simulink model "motor_sensorless"  (R2020a)
settings: Solver=FixedStepDiscrete  StartTime=0.0  StopTime=inf  FixedStep=ts  RelTol=1e-3
values from neighbouring files (symbols this model uses):
  adgain_and_ivscale = round(0.33*1.56*4096/3.3*SC_SCALE/IV_SCALE)    [def_param.m]
  cos23z = round(cos(2.0/3.0*pi)*sqrt(2.0/3.0)*SC_SCALE)    [def_param.m]
  cos43z = round(cos(4.0/3.0*pi)*sqrt(2.0/3.0)*SC_SCALE)    [def_param.m]
  COUNT2RPM = round(FS/SC_SCALE*60/7)    [def_param.m]
  DUTY2VOLT = round(VCC*IV_SCALE/MAX_PWM_DUTY)    [def_param.m]
  FF_CURRENT = 1500    [def_param.m]
  FS = 20000    [def_param.m]
  iKi_pll = round(1/Ki_pll)    [def_param.m]
  iKp_curr_d = iKp_curr    [def_param.m]
  iKp_curr_q = iKp_curr    [def_param.m]
  iKp_pll = round(1/Kp_pll)    [def_param.m]
  Ki_curr_d = Ki_curr    [def_param.m]
  Ki_curr_q = Ki_curr    [def_param.m]
  Kp_velo = 5    [def_param.m]
  Ra_scale = round(Ra*SC_SCALE)    [def_param.m]
  SC_SCALE = 32768    [def_param.m]
  sin23z = round(sin(2.0/3.0*pi)*sqrt(2.0/3.0)*SC_SCALE)    [def_param.m]
  sin43z = round(sin(4.0/3.0*pi)*sqrt(2.0/3.0)*SC_SCALE)    [def_param.m]
  sqrt23 = round(sqrt(2.0/3.0)*SC_SCALE)    [def_param.m]
libraries: simulink x2, arduinolib x1
settings Model: SimulationMode=external  SILPILModeSetting=veronly  ExtModeTrigDuration=1  Creator=hirata  LastModifiedBy=hirata
settings DataIOCC: SaveOutput=off  SignalLogging=off  DSMLogging=off  SaveTime=off  ReturnWorkspaceOutputs=off
settings OptimizationCC: EnhancedBackFolding=on  PassReuseOutputArgsAs=Individual arguments  ZeroExternalMemoryAtStartup=off  ZeroInternalMemoryAtStartup=off  MaxStackSize=64  OptimizeBlockOrder=speed  DifferentSizesBufferReuse=on  OptimizationCustomize=off  EfficientTunableParamExpr=on
settings DebuggingCC: MultiTaskDSMMsg=none  ParameterTunabilityLossMsg=error
settings HardwareCC: ProdBitPerPointer=32  ProdBitPerSizeT=32  ProdBitPerPtrDiffT=32  ProdLargestAtomicInteger=Long  ProdLargestAtomicFloat=Double  ProdWordSize=32  ProdHWDeviceType=ARM Compatible->ARM Cortex  UseEmbeddedCoderFeatures=off  UseSimulinkCoderFeatures=off
settings SFSimCC: MATLABDynamicMemAlloc=off
settings RTWCC: SystemTargetFile=ert.tlc  HardwareBoard=Arduino Due  TLCOptions=-aInlineSetEventsForThisBaseRateFcn=TLC_FALSE -aSuppressMultiTaskScheduler=TLC_FALSE -aRateBasedStepFcn=1  TemplateMakefile=ert_default_tmf  Toolchain=Arduino ARM  BuildConfiguration=Faster Runs
settings CodeAppCC: ForceParamTrailComments=on  IgnoreCustomStorageClasses=off  OperatorAnnotations=on  SimulinkDataObjDesc=on  SFDataObjDesc=on  InsertBlockDesc=on
settings ERTTargetCC: SupportContinuousTime=on  SupportNonInlinedSFcns=on  SupportVariableSizeSignals=on  ExtModeStaticAllocSize=24576

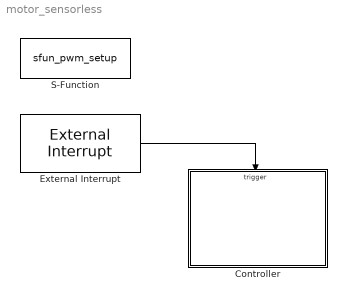
== system motor_sensorless ==
  Controller : Subsystem
  External Interrupt : arduinolib/External Interrupt  Pin=2  PullUp=off  Mode=RISING  InterruptSimulationInput=off
      settings: SourceProductBaseCode=ARDUINO
  S-Function : S-Function  FunctionName=sfun_pwm_setup  SFunctionDeploymentMode=off  EnableBusSupport=off
  wires:
  External Interrupt/1 -> Controller/Trigger

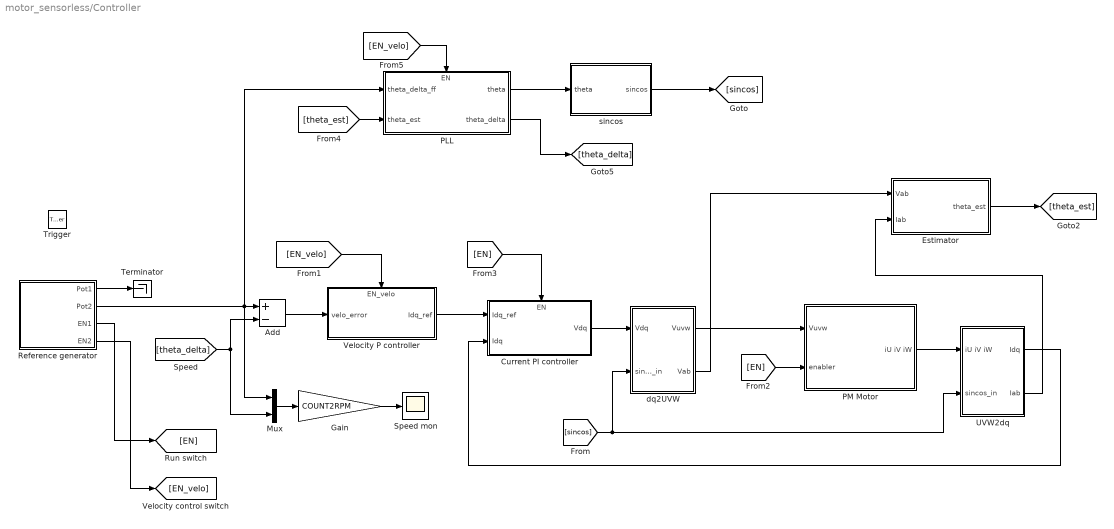
== system motor_sensorless/Controller ==
  Trigger : TriggerPort  TriggerType=function-call  VariantControl=Variant  PortDimensions=1
  Add : Sum  Inputs=+-
  Current PI controller : Subsystem
      settings: PortSchema="{\"entries\":[{\"content\":{\"sides\":[{\"content\":{\"connectorIds\":[\"In1\",\"In2\"]},\"type\":\"ConnectorPlacement.EquallySpacedRectSide\",\"uuid\":\"51bdd515-79d8-44f5-b943-076c1de5691d\"},{\"content\":{\"connectorIds\":[\"Out1\"],\"side\":\"RIGHT\"},\"type\":\"ConnectorPlacement.EquallySpacedRectSide\",\"uuid\":\"02ded229-b196-46a0-b1f1-559478ee2a5f\"},{\"content\":{\"connectorIds\":[\"In3\"],\"side\":\"TOP\"},\"type\":\"ConnectorPlacement.EquallySpacedRectSide\",\"uuid\":\"45d1ca2d-8d37-43f9-8461-d73100be391d\"}]},\"type\":\"ConnectorPlacement.EquallySpacedConnector\",\"uuid\":\"0325882b-c054-4400-b3a7-6975fb1af6b3\"}],\"packageUris\":[\"http://schema.mathworks.com/mf0/Connector/19700101\"],\"version\":\"1.0\"}"
  Estimator : Subsystem
  Gain : Gain  Gain=COUNT2RPM  ParamDataTypeStr=int32  OutDataTypeStr=int32
  Mux : Mux  Inputs=2
  PLL : Subsystem
      settings: PortSchema="{\"entries\":[{\"content\":{\"sides\":[{\"content\":{\"connectorIds\":[\"In1\",\"In2\"]},\"type\":\"ConnectorPlacement.EquallySpacedRectSide\",\"uuid\":\"c1279200-642a-4817-bff2-49f1fc45cae9\"},{\"content\":{\"connectorIds\":[\"Out1\",\"Out2\"],\"side\":\"RIGHT\"},\"type\":\"ConnectorPlacement.EquallySpacedRectSide\",\"uuid\":\"60873783-c9ec-4a70-a078-e4f3fd5ab03e\"},{\"content\":{\"connectorIds\":[\"In3\"],\"side\":\"TOP\"},\"type\":\"ConnectorPlacement.EquallySpacedRectSide\",\"uuid\":\"f4a28572-fe2d-4ee0-bb44-94978f18e4bd\"}]},\"type\":\"ConnectorPlacement.EquallySpacedConnector\",\"uuid\":\"bfaa0106-d9f2-4ecc-a1fc-3a6fb0b4180b\"}],\"packageUris\":[\"http://schema.mathworks.com/mf0/Connector/19700101\"],\"version\":\"1.0\"}"
  PM Motor : Subsystem
  Reference generator : Subsystem
  Speed mon : Scope
  Terminator : Terminator
  UVW2dq : Subsystem
  Velocity P controller : Subsystem
      settings: PortSchema="{\"entries\":[{\"content\":{\"sides\":[{\"content\":{\"connectorIds\":[\"In1\"]},\"type\":\"ConnectorPlacement.EquallySpacedRectSide\",\"uuid\":\"ec985efa-ceb5-40b6-8715-0b6e8d029389\"},{\"content\":{\"connectorIds\":[\"Out1\"],\"side\":\"RIGHT\"},\"type\":\"ConnectorPlacement.EquallySpacedRectSide\",\"uuid\":\"25d854cf-6db0-4509-b167-323bc7ab570a\"},{\"content\":{\"connectorIds\":[\"In2\"],\"side\":\"TOP\"},\"type\":\"ConnectorPlacement.EquallySpacedRectSide\",\"uuid\":\"c6db0138-fa8b-40e2-8338-1c9cb4bbe622\"}]},\"type\":\"ConnectorPlacement.EquallySpacedConnector\",\"uuid\":\"967c00c6-7ce0-4d1f-a7f0-366bbe0d8034\"}],\"packageUris\":[\"http://schema.mathworks.com/mf0/Connector/19700101\"],\"version\":\"1.0\"}"
  dq2UVW : Subsystem
  sincos : Subsystem
  wires:
  dq2UVW/1(Vuvw) -> PM Motor/1(Vuvw)
  [sincos] -> dq2UVW/2(sincos_in), UVW2dq/2(sincos_in)
  PM Motor/1(iU iV iW) -> UVW2dq/1(iU iV iW)
  UVW2dq/1(Idq) -> Current PI controller/2(Idq)
  [EN] -> PM Motor/2(enabler)
  Current PI controller/1(Vdq) -> dq2UVW/1(Vdq)
  [EN] -> Current PI controller/3(EN)
  dq2UVW/2(Vab) -> Estimator/1(Vab)
  UVW2dq/2(Iab) -> Estimator/2(Iab)
  Estimator/1(theta_est) -> [theta_est]
  [theta_est] -> PLL/2(theta_est)
  [EN_velo] -> PLL/3(EN)
  PLL/1(theta) -> sincos/1(theta)
  sincos/1(sincos) -> [sincos]
  Add/1 -> Velocity P controller/1(velo_error)
  [EN_velo] -> Velocity P controller/2(EN_velo)
  Velocity P controller/1(Idq_ref) -> Current PI controller/1(Idq_ref)
  PLL/2(theta_delta) -> [theta_delta]
  [theta_delta] -> Mux/2, Add/2
  Reference generator/2(Pot2) -> Mux/1, PLL/1(theta_delta_ff), Add/1
  Reference generator/3(EN1) -> [EN]
  Reference generator/4(EN2) -> [EN_velo]
  Mux/1 -> Gain/1
  Reference generator/1(Pot1) -> Terminator/1
  Gain/1 -> Speed mon/1

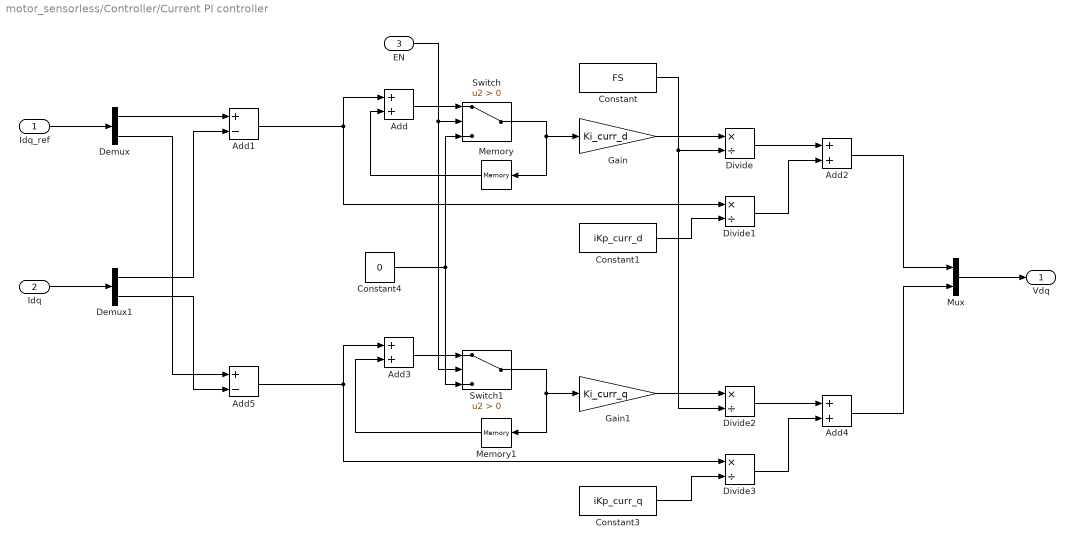
== system motor_sensorless/Controller/Current PI controller ==
  Idq_ref : Inport
  Idq : Inport  Port=2
  EN : Inport  Port=3
  Add{,2..4} (4 alike) : Sum
  Add1 : Sum  Inputs=+-
  Add5 : Sum  Inputs=+-
  Constant : Constant  Value=FS  OutDataTypeStr=int32
  Constant1 : Constant  Value=iKp_curr_d  OutDataTypeStr=int32
  Constant3 : Constant  Value=iKp_curr_q  OutDataTypeStr=int32
  Constant4 : Constant  Value=0  OutDataTypeStr=int32
  Demux : Demux  Outputs=2
  Demux1 : Demux  Outputs=2
  Divide{,1..3} (4 alike) : Product  Inputs=*/
  Gain : Gain  Gain=Ki_curr_d  ParamDataTypeStr=int32  OutDataTypeStr=int32
  Gain1 : Gain  Gain=Ki_curr_q  ParamDataTypeStr=int32  OutDataTypeStr=int32
  Memory : Memory  InheritSampleTime=on
  Memory1 : Memory  InheritSampleTime=on
  Mux : Mux  Inputs=2
  Switch : Switch  Criteria=u2 > Threshold  OutDataTypeStr=int32
  Switch1 : Switch  Criteria=u2 > Threshold  OutDataTypeStr=int32
  Vdq : Outport
  wires:
  Memory/1 -> Add/2
  Switch/1 -> Memory/1, Gain/1
  Add1/1 -> Add/1, Divide1/1
  Gain/1 -> Divide/1
  Constant1/1 -> Divide1/2
  Divide/1 -> Add2/1
  Divide1/1 -> Add2/2
  Gain1/1 -> Divide2/1
  Add5/1 -> Add3/1, Divide3/1
  Switch1/1 -> Memory1/1, Gain1/1
  Memory1/1 -> Add3/2
  Divide3/1 -> Add4/2
  Constant3/1 -> Divide3/2
  Constant/1 -> Divide/2, Divide2/2
  Divide2/1 -> Add4/1
  Add2/1 -> Mux/1
  Mux/1 -> Vdq/1
  Add4/1 -> Mux/2
  Idq/1 -> Demux1/1
  Idq_ref/1 -> Demux/1
  Demux/1 -> Add1/1
  Demux/2 -> Add5/1
  Demux1/1 -> Add1/2
  Demux1/2 -> Add5/2
  Add/1 -> Switch/1
  Add3/1 -> Switch1/1
  EN/1 -> Switch1/2, Switch/2
  Constant4/1 -> Switch1/3, Switch/3

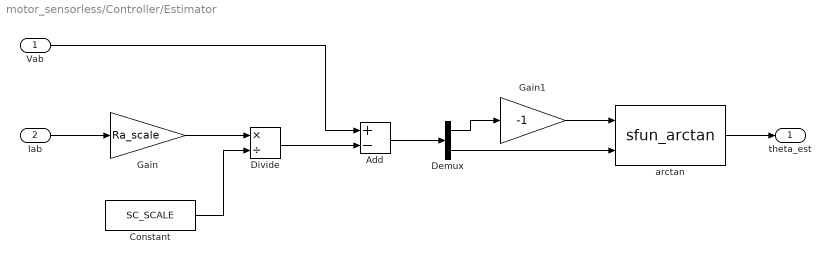
== system motor_sensorless/Controller/Estimator ==
  Vab : Inport
  Iab : Inport  Port=2
  Add : Sum  Inputs=+-
  Constant : Constant  Value=SC_SCALE  OutDataTypeStr=int32
  Demux : Demux  Outputs=2
  Divide : Product  Inputs=*/
  Gain : Gain  Gain=Ra_scale  ParamDataTypeStr=int32  OutDataTypeStr=int32
  Gain1 : Gain  Gain=-1  ParamDataTypeStr=int32  OutDataTypeStr=int32
  arctan : S-Function  FunctionName=sfun_arctan  SFunctionDeploymentMode=off  EnableBusSupport=off
  theta_est : Outport
  wires:
  arctan/1 -> theta_est/1
  Gain/1 -> Divide/1
  Constant/1 -> Divide/2
  Iab/1 -> Gain/1
  Divide/1 -> Add/2
  Vab/1 -> Add/1
  Gain1/1 -> arctan/1
  Add/1 -> Demux/1
  Demux/1 -> Gain1/1
  Demux/2 -> arctan/2

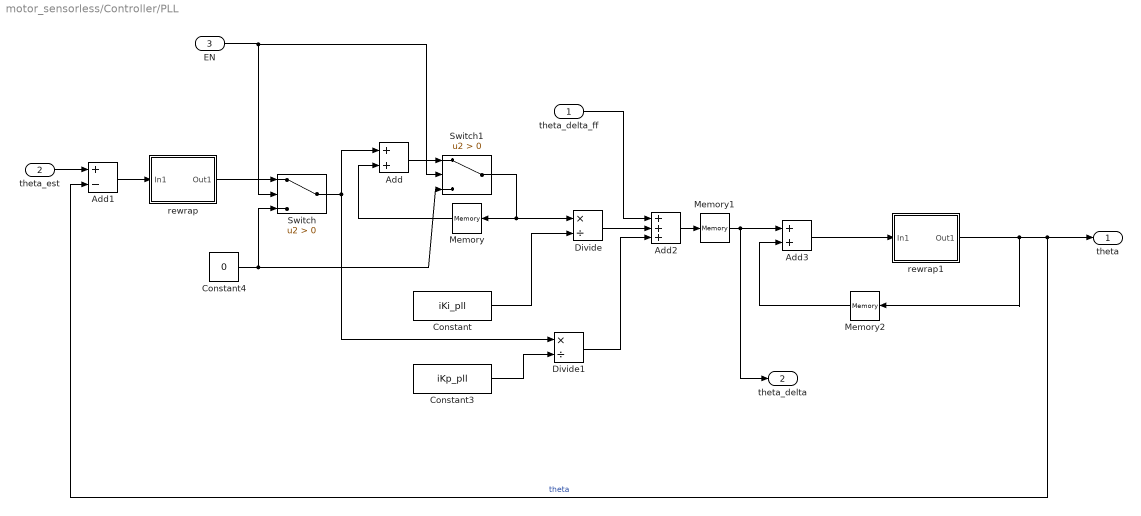
== system motor_sensorless/Controller/PLL ==
  theta_delta_ff : Inport
  theta_est : Inport  Port=2
  EN : Inport  Port=3
  Add : Sum
  Add1 : Sum  Inputs=+-
  Add2 : Sum  Inputs=+++
  Add3 : Sum
  Constant : Constant  Value=iKi_pll  OutDataTypeStr=int32
  Constant3 : Constant  Value=iKp_pll  OutDataTypeStr=int32
  Constant4 : Constant  Value=0  OutDataTypeStr=int32
  Divide : Product  Inputs=*/
  Divide1 : Product  Inputs=*/
  Memory : Memory  InheritSampleTime=on
  Memory1 : Memory  InheritSampleTime=on
  Memory2 : Memory  InheritSampleTime=on
  Switch : Switch  Criteria=u2 > Threshold  OutDataTypeStr=int32
  Switch1 : Switch  Criteria=u2 > Threshold  OutDataTypeStr=int32
  rewrap : Subsystem
  rewrap1 : Subsystem
  theta : Outport
  theta_delta : Outport  Port=2
  wires:
  Constant3/1 -> Divide1/2
  Divide/1 -> Add2/2
  Switch1/1 -> Divide/1, Memory/1
  EN/1 -> Switch/2, Switch1/2
  Memory/1 -> Add/2
  Constant/1 -> Divide/2
  Divide1/1 -> Add2/3
  Constant4/1 -> Switch/3, Switch1/3
  Switch/1 -> Add/1, Divide1/1
  theta_est/1 -> Add1/1
  rewrap1/1(Out1) -> Memory2/1, theta/1, Add1/2  "theta"
  theta_delta_ff/1 -> Add2/1
  Add1/1 -> rewrap/1(In1)
  rewrap/1(Out1) -> Switch/1
  Add/1 -> Switch1/1
  Add2/1 -> Memory1/1
  Add3/1 -> rewrap1/1(In1)
  Memory1/1 -> Add3/1, theta_delta/1
  Memory2/1 -> Add3/2

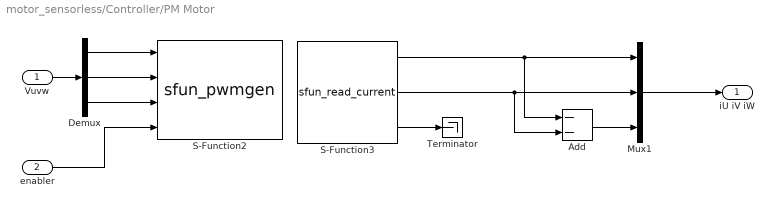
== system motor_sensorless/Controller/PM Motor ==
  Vuvw : Inport
  enabler : Inport  Port=2
  Add : Sum  Inputs=--
  Demux : Demux  Outputs=3
  Mux1 : Mux  Inputs=3
  S-Function2 : S-Function  FunctionName=sfun_pwmgen  SFunctionDeploymentMode=off  EnableBusSupport=off
  S-Function3 : S-Function  FunctionName=sfun_read_current  SFunctionDeploymentMode=off  EnableBusSupport=off
  Terminator : Terminator
  iU iV iW : Outport
  wires:
  Demux/1 -> S-Function2/1
  Vuvw/1 -> Demux/1
  Demux/2 -> S-Function2/2
  Demux/3 -> S-Function2/3
  enabler/1 -> S-Function2/4
  Mux1/1 -> iU iV iW/1
  S-Function3/1 -> Add/1, Mux1/1
  S-Function3/2 -> Add/2, Mux1/2
  S-Function3/3 -> Terminator/1
  Add/1 -> Mux1/3

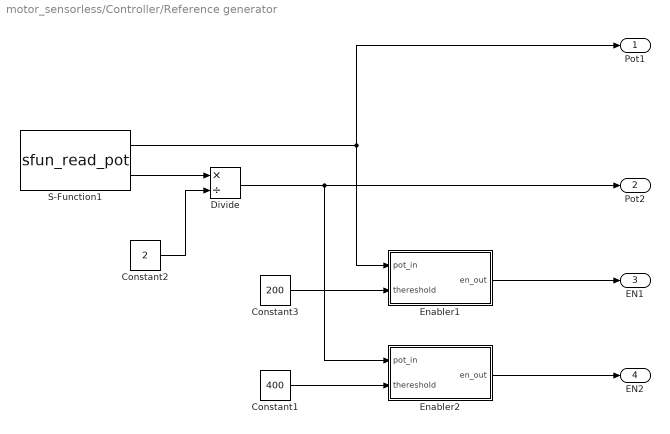
== system motor_sensorless/Controller/Reference generator ==
  Constant1 : Constant  Value=400  OutDataTypeStr=int32
  Constant2 : Constant  Value=2  OutDataTypeStr=int32
  Constant3 : Constant  Value=200  OutDataTypeStr=int32
  Divide : Product  Inputs=*/  OutDataTypeStr=int32
  Enabler1 : Subsystem
  Enabler2 : Subsystem
  S-Function1 : S-Function  FunctionName=sfun_read_pot  SFunctionDeploymentMode=off  EnableBusSupport=off
  Pot1 : Outport
  Pot2 : Outport  Port=2
  EN1 : Outport  Port=3
  EN2 : Outport  Port=4
  wires:
  S-Function1/1 -> Pot1/1, Enabler1/1(pot_in)
  Enabler2/1(en_out) -> EN2/1
  Divide/1 -> Enabler2/1(pot_in), Pot2/1
  Enabler1/1(en_out) -> EN1/1
  Constant3/1 -> Enabler1/2(thereshold)
  Constant1/1 -> Enabler2/2(thereshold)
  S-Function1/2 -> Divide/1
  Constant2/1 -> Divide/2

== system motor_sensorless/Controller/UVW2dq ==
  iU iV iW : Inport
  sincos_in : Inport  Port=2
  Demux : Demux  Outputs=3
  Mux : Mux  Inputs=2
  UVW2ab : Subsystem
  ab2dq : Subsystem
  Idq : Outport
  Iab : Outport  Port=2
  wires:
  UVW2ab/2(Ib) -> Mux/2, ab2dq/2(b_in)
  Demux/1 -> UVW2ab/1(U)
  UVW2ab/1(Ia) -> Mux/1, ab2dq/1(a_in)
  Demux/2 -> UVW2ab/2(V)
  ab2dq/1(dq_out) -> Idq/1
  Demux/3 -> UVW2ab/3(W)
  sincos_in/1 -> ab2dq/3(sincos_in)
  iU iV iW/1 -> Demux/1
  Mux/1 -> Iab/1

== system motor_sensorless/Controller/Velocity P controller ==
  velo_error : Inport
  EN_velo : Inport  Port=2
  Constant1 : Constant  Value=0  OutDataTypeStr=int32
  Constant4 : Constant  Value=FF_CURRENT  OutDataTypeStr=int32
  Gain : Gain  Gain=Kp_velo  ParamDataTypeStr=int32  OutDataTypeStr=int32
  Mux : Mux  Inputs=2
  Switch : Switch  Criteria=u2 > Threshold  OutDataTypeStr=int32
  Idq_ref : Outport
  wires:
  Switch/1 -> Mux/2
  Constant1/1 -> Mux/1
  Constant4/1 -> Switch/3
  EN_velo/1 -> Switch/2
  Gain/1 -> Switch/1
  velo_error/1 -> Gain/1
  Mux/1 -> Idq_ref/1

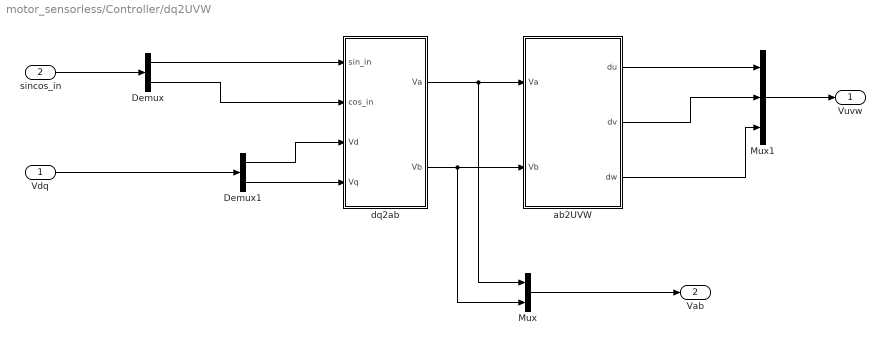
== system motor_sensorless/Controller/dq2UVW ==
  Vdq : Inport
  sincos_in : Inport  Port=2
  Demux : Demux  Outputs=2
  Demux1 : Demux  Outputs=2
  Mux : Mux  Inputs=2
  Mux1 : Mux  Inputs=3
  ab2UVW : Subsystem
  dq2ab : Subsystem
  Vuvw : Outport
  Vab : Outport  Port=2
  wires:
  dq2ab/2(Vb) -> Mux/2, ab2UVW/2(Vb)
  dq2ab/1(Va) -> Mux/1, ab2UVW/1(Va)
  Demux1/2 -> dq2ab/4(Vq)
  ab2UVW/1(du) -> Mux1/1
  sincos_in/1 -> Demux/1
  Demux/1 -> dq2ab/1(sin_in)
  Demux/2 -> dq2ab/2(cos_in)
  Mux/1 -> Vab/1
  ab2UVW/2(dv) -> Mux1/2
  ab2UVW/3(dw) -> Mux1/3
  Mux1/1 -> Vuvw/1
  Demux1/1 -> dq2ab/3(Vd)
  Vdq/1 -> Demux1/1

== system motor_sensorless/Controller/sincos ==
  theta : Inport
  Mux : Mux  Inputs=2
  S-Function2 : S-Function  FunctionName=sfun_sincos  SFunctionDeploymentMode=off  EnableBusSupport=off
  sincos : Outport
  wires:
  S-Function2/2 -> Mux/2
  S-Function2/1 -> Mux/1
  Mux/1 -> sincos/1
  theta/1 -> S-Function2/1

== system motor_sensorless/Controller/PLL/rewrap ==
  In1 : Inport
  Add : Sum
  Add1 : Sum  Inputs=-+
  Bitwise Operator3 : simulink/Logic and Bit Operations/Bitwise Operator  logicop=AND  UseBitMask=on  BitMask=0x7FFF  BitMaskRealWorld=Stored Integer
  Constant : Constant  Value=16384  OutDataTypeStr=int32
  Out1 : Outport
  wires:
  Bitwise Operator3/1 -> Add1/2
  In1/1 -> Add/2
  Constant/1 -> Add1/1, Add/1
  Add/1 -> Bitwise Operator3/1
  Add1/1 -> Out1/1

== system motor_sensorless/Controller/PLL/rewrap1 ==
  In1 : Inport
  Add : Sum
  Add1 : Sum  Inputs=-+
  Bitwise Operator3 : simulink/Logic and Bit Operations/Bitwise Operator  logicop=AND  UseBitMask=on  BitMask=0x7FFF  BitMaskRealWorld=Stored Integer
  Constant : Constant  Value=16384  OutDataTypeStr=int32
  Out1 : Outport
  wires:
  Bitwise Operator3/1 -> Add1/2
  In1/1 -> Add/2
  Constant/1 -> Add1/1, Add/1
  Add/1 -> Bitwise Operator3/1
  Add1/1 -> Out1/1

== system motor_sensorless/Controller/Reference generator/Enabler1 ==
  pot_in : Inport
  thereshold : Inport  Port=2
  Data Type Conversion : DataTypeConversion  OutDataTypeStr=int32
  Relational Operator : RelationalOperator  Operator=>  OutDataTypeStr=boolean  RndMeth=Simplest
  en_out : Outport
  wires:
  Relational Operator/1 -> Data Type Conversion/1
  Data Type Conversion/1 -> en_out/1
  thereshold/1 -> Relational Operator/2
  pot_in/1 -> Relational Operator/1

== system motor_sensorless/Controller/Reference generator/Enabler2 ==
  pot_in : Inport
  thereshold : Inport  Port=2
  Data Type Conversion : DataTypeConversion  OutDataTypeStr=int32
  Relational Operator : RelationalOperator  Operator=>  OutDataTypeStr=boolean  RndMeth=Simplest
  en_out : Outport
  wires:
  pot_in/1 -> Relational Operator/1
  thereshold/1 -> Relational Operator/2
  Data Type Conversion/1 -> en_out/1
  Relational Operator/1 -> Data Type Conversion/1

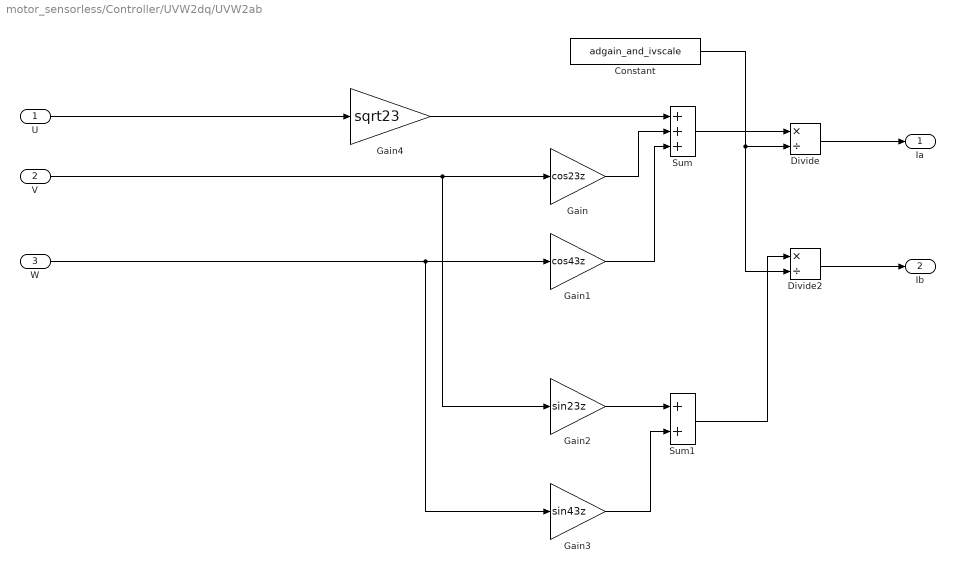
== system motor_sensorless/Controller/UVW2dq/UVW2ab ==
  U : Inport
  V : Inport  Port=2
  W : Inport  Port=3
  Constant : Constant  Value=adgain_and_ivscale  OutDataTypeStr=int32
  Divide : Product  Inputs=*/  OutDataTypeStr=int32
  Divide2 : Product  Inputs=*/  OutDataTypeStr=int32
  Gain : Gain  Gain=cos23z  ParamDataTypeStr=int32  OutDataTypeStr=int32
  Gain1 : Gain  Gain=cos43z  ParamDataTypeStr=int32  OutDataTypeStr=int32
  Gain2 : Gain  Gain=sin23z  ParamDataTypeStr=int32  OutDataTypeStr=int32
  Gain3 : Gain  Gain=sin43z  ParamDataTypeStr=int32  OutDataTypeStr=int32
  Gain4 : Gain  Gain=sqrt23  ParamDataTypeStr=int32  OutDataTypeStr=int32
  Sum : Sum  Inputs=+++  AccumDataTypeStr=int32  OutDataTypeStr=int32
  Sum1 : Sum  AccumDataTypeStr=int32  OutDataTypeStr=int32
  Ia : Outport
  Ib : Outport  Port=2
  wires:
  U/1 -> Gain4/1
  Gain/1 -> Sum/2
  Gain1/1 -> Sum/3
  Gain3/1 -> Sum1/2
  Gain2/1 -> Sum1/1
  V/1 -> Gain2/1, Gain/1
  W/1 -> Gain3/1, Gain1/1
  Gain4/1 -> Sum/1
  Constant/1 -> Divide2/2, Divide/2
  Sum/1 -> Divide/1
  Divide/1 -> Ia/1
  Divide2/1 -> Ib/1
  Sum1/1 -> Divide2/1

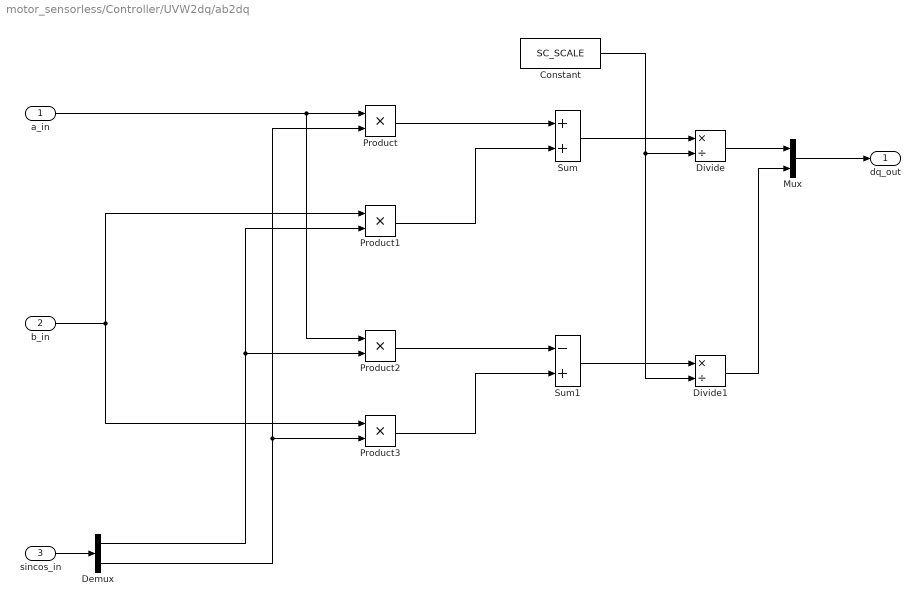
== system motor_sensorless/Controller/UVW2dq/ab2dq ==
  a_in : Inport
  b_in : Inport  Port=2
  sincos_in : Inport  Port=3
  Constant : Constant  Value=SC_SCALE  OutDataTypeStr=int32
  Demux : Demux  Outputs=2
  Divide : Product  Inputs=*/  OutDataTypeStr=int32
  Divide1 : Product  Inputs=*/  OutDataTypeStr=int32
  Mux : Mux  Inputs=2
  Product{,1..3} (4 alike) : Product  OutDataTypeStr=int32
  Sum : Sum
  Sum1 : Sum  Inputs=-+
  dq_out : Outport
  wires:
  a_in/1 -> Product2/1, Product/1
  Product/1 -> Sum/1
  Product1/1 -> Sum/2
  b_in/1 -> Product3/1, Product1/1
  Demux/2 -> Product3/2, Product/2
  Demux/1 -> Product2/2, Product1/2
  Product2/1 -> Sum1/1
  Product3/1 -> Sum1/2
  sincos_in/1 -> Demux/1
  Constant/1 -> Divide1/2, Divide/2
  Sum1/1 -> Divide1/1
  Sum/1 -> Divide/1
  Divide/1 -> Mux/1
  Divide1/1 -> Mux/2
  Mux/1 -> dq_out/1

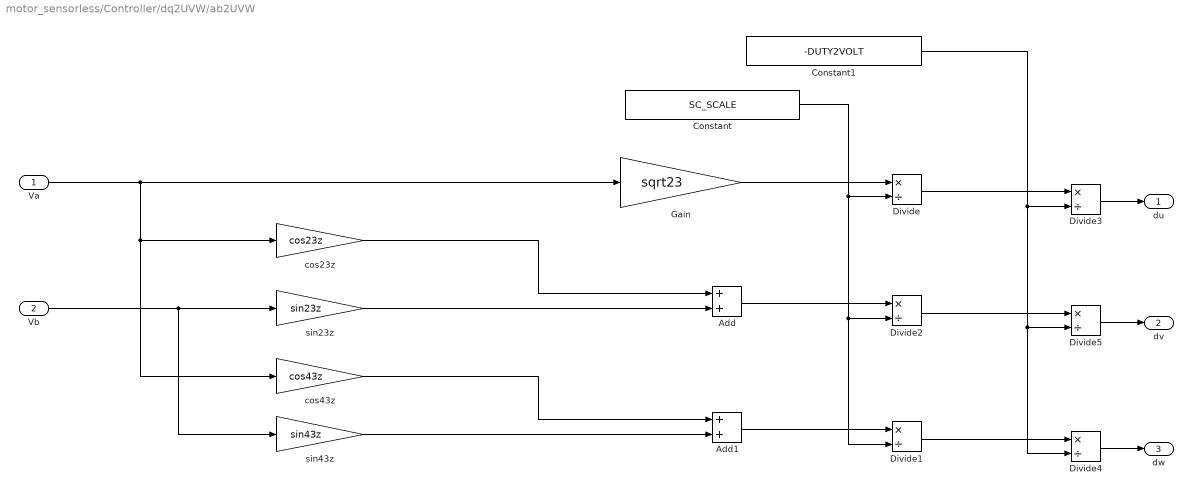
== system motor_sensorless/Controller/dq2UVW/ab2UVW ==
  Va : Inport
  Vb : Inport  Port=2
  Add : Sum
  Add1 : Sum
  Constant : Constant  Value=SC_SCALE  OutDataTypeStr=int32
  Constant1 : Constant  Value=-DUTY2VOLT  OutDataTypeStr=int32
  Divide{,1..5} (6 alike) : Product  Inputs=*/  OutDataTypeStr=int32
  Gain : Gain  Gain=sqrt23  ParamDataTypeStr=int32  OutDataTypeStr=int32
  cos23z : Gain  Gain=cos23z  ParamDataTypeStr=int32  OutDataTypeStr=int32
  cos43z : Gain  Gain=cos43z  ParamDataTypeStr=int32  OutDataTypeStr=int32
  sin23z : Gain  Gain=sin23z  ParamDataTypeStr=int32  OutDataTypeStr=int32
  sin43z : Gain  Gain=sin43z  ParamDataTypeStr=int32  OutDataTypeStr=int32
  du : Outport
  dv : Outport  Port=2
  dw : Outport  Port=3
  wires:
  Gain/1 -> Divide/1
  Add1/1 -> Divide1/1
  Va/1 -> Gain/1, cos43z/1, cos23z/1
  Vb/1 -> sin43z/1, sin23z/1
  cos23z/1 -> Add/1
  sin23z/1 -> Add/2
  sin43z/1 -> Add1/2
  cos43z/1 -> Add1/1
  Add/1 -> Divide2/1
  Constant/1 -> Divide1/2, Divide2/2, Divide/2
  Divide2/1 -> Divide5/1
  Constant1/1 -> Divide4/2, Divide5/2, Divide3/2
  Divide1/1 -> Divide4/1
  Divide/1 -> Divide3/1
  Divide3/1 -> du/1
  Divide5/1 -> dv/1
  Divide4/1 -> dw/1

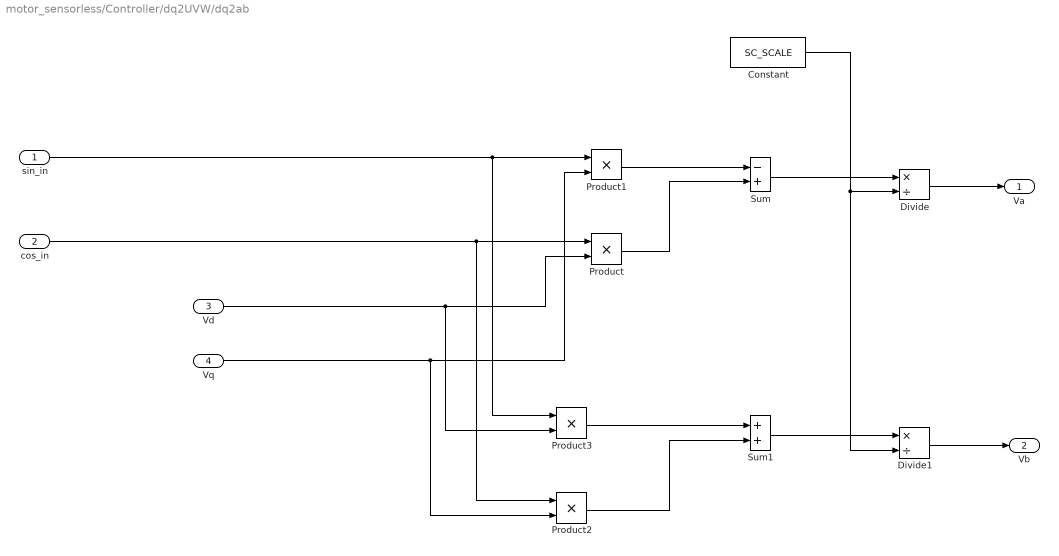
== system motor_sensorless/Controller/dq2UVW/dq2ab ==
  sin_in : Inport
  cos_in : Inport  Port=2
  Vd : Inport  Port=3
  Vq : Inport  Port=4
  Constant : Constant  Value=SC_SCALE  OutDataTypeStr=int32
  Divide : Product  Inputs=*/  OutDataTypeStr=int32
  Divide1 : Product  Inputs=*/  OutDataTypeStr=int32
  Product{,1..3} (4 alike) : Product  OutDataTypeStr=int32
  Sum : Sum  Inputs=-+
  Sum1 : Sum
  Va : Outport
  Vb : Outport  Port=2
  wires:
  cos_in/1 -> Product2/1, Product/1
  Vd/1 -> Product3/2, Product/2
  sin_in/1 -> Product1/1, Product3/1
  Vq/1 -> Product2/2, Product1/2
  Product1/1 -> Sum/1
  Product/1 -> Sum/2
  Sum/1 -> Divide/1
  Product3/1 -> Sum1/1
  Sum1/1 -> Divide1/1
  Product2/1 -> Sum1/2
  Divide/1 -> Va/1
  Divide1/1 -> Vb/1
  Constant/1 -> Divide1/2, Divide/2
